simulink subsystem "PvtSubSys_VSM_ELK"  (R2020b)
settings: Solver=VariableStepAuto  StartTime=0.0  StopTime=10.0  RelTol=1e-3
values from neighbouring files (symbols this model uses):
  P_VSM_ELK_Curvature_R_Table : value not decoded    [ELK.sldd]
  P_VSM_ELK_Curvature_R_Table_Calibration : value not decoded    [ELK.sldd]
  P_VSM_ELK_Lane_Width_Table : value not decoded    [ELK.sldd]
  P_VSM_ELK_Lane_Width_Table_Calibration : value not decoded    [ELK.sldd]
  P_VSM_ELK_Lateral_Speed_Table : value not decoded    [ELK.sldd]
  P_VSM_ELK_Lateral_Speed_Table_Calibration : value not decoded    [ELK.sldd]
  P_VSM_ELK_OnComing_Lateral = 2.8    [ELK.sldd]
  P_VSM_ELK_OnComing_TTC = 3.0    [ELK.sldd]
  P_VSM_ELK_OverTaking_Lateral = 2.0    [ELK.sldd]
  P_VSM_ELK_OverTaking_TTC = 5.0    [ELK.sldd]
  P_VSM_ELK_Sensitive_Table : value not decoded    [ELK.sldd]
  P_VSM_ELK_Sensitive_Table_Calibration : value not decoded    [ELK.sldd]
  P_VSM_ELK_State_Absesp_enable = 1.0    [ELK.sldd]
  P_VSM_ELK_State_Accpedalrate_enable = 1.0    [ELK.sldd]
  P_VSM_ELK_State_Breakpressure_enable = 1.0    [ELK.sldd]
  P_VSM_ELK_State_DriverInputTrqValue_enable = 1.0    [ELK.sldd]
  P_VSM_ELK_State_Eps_enable = 1.0    [ELK.sldd]
  P_VSM_ELK_State_ESSSts_enable = 1.0    [ELK.sldd]
  P_VSM_ELK_State_Failsafe_enable = 1.0    [ELK.sldd]
  P_VSM_ELK_State_GEAR_enable = 1.0    [ELK.sldd]
  P_VSM_ELK_State_Handson_enable = 1.0    [ELK.sldd]
  P_VSM_ELK_State_Headingangle_enable = 1.0    [ELK.sldd]
  P_VSM_ELK_State_Lane_enable = 1.0    [ELK.sldd]
  P_VSM_ELK_State_LaneChange_enable = 1.0    [ELK.sldd]
  P_VSM_ELK_State_Lanecurve_enable = 1.0    [ELK.sldd]
  P_VSM_ELK_State_LateralAcce_enable = 1.0    [ELK.sldd]
  P_VSM_ELK_State_LongitudeAcc_enable = 1.0    [ELK.sldd]
  P_VSM_ELK_State_Overide_enable = 1.0    [ELK.sldd]
  P_VSM_ELK_State_Param_AngleOffset = 0.05    [ELK.sldd]
  P_VSM_ELK_State_Param_LaneTime : value not decoded    [ELK.sldd]
  P_VSM_ELK_State_Param_Oncoming = 0.55    [ELK.sldd]
  P_VSM_ELK_State_Param_OnTime : value not decoded    [ELK.sldd]
  P_VSM_ELK_State_Param_OutOffset = 0.15    [ELK.sldd]
  P_VSM_ELK_State_Param_Over = 0.55    [ELK.sldd]
  P_VSM_ELK_State_Param_OvTime : value not decoded    [ELK.sldd]
  P_VSM_ELK_State_Param_Speed : value not decoded    [ELK.sldd]
  P_VSM_ELK_State_SteerWheelAngle_enable = 1.0    [ELK.sldd]
  P_VSM_ELK_State_SteerWheelSpd_enable = 1.0    [ELK.sldd]
  P_VSM_ELK_State_TurnLight_enable = 1.0    [ELK.sldd]
  P_VSM_ELK_State_Vehspeed_enable = 1.0    [ELK.sldd]
  P_VSM_ELK_State_Yawsup_enable = 1.0    [ELK.sldd]
undefined symbols (not defined in the file or in its folder): ELKSTATE, P_Global_DxvRearBumper_m, P_Global_IEnvironment_RefPX_Front_Bumper, P_Global_IFV2Fwheel_Dx, P_Global_Vehicle_Length_m, P_Global_VehicleWidthMin_m, P_VSM_LSMC_SampleTime
libraries: simulink x167
(part 1 of 5)
settings Model: Creator=GW00133806  LastModifiedBy=GW00199575

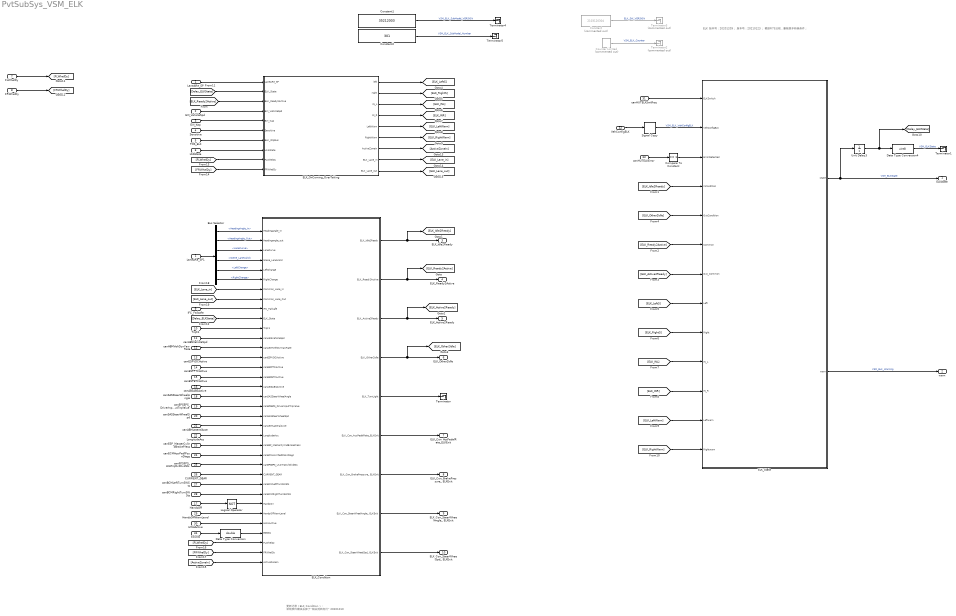
== system PvtSubSys_VSM_ELK ==
  note: 更新记录（ELK_Condition）：
      | 常规条件模块去掉了“相关则转向灯”
      | 20201010
  note: ELK
      | 版本号：20201209；
      | 版本号：20210123；
      | 根据R79法规，删除脱手转换条件；
  LaneARe_SP : Inport  OutDataTypeStr=Bus: LaneARe_SP
  EVI_VehicleSpd : Inport  Port=2  OutDataTypeStr=single
  EVI_Kap : Inport  Port=3  OutDataTypeStr=single
  Sensitive : Inport  Port=4  OutDataTypeStr=uint8
  TOS_ELK : Inport  Port=5  OutDataTypeStr=Bus: TOS_ELK_BUS  BusOutputAsStruct=on
  LKAState : Inport  Port=6  OutDataTypeStr=uint8
  FLWhelDy : Inport  Port=7  OutDataTypeStr=single
  FRWhelDy : Inport  Port=8  OutDataTypeStr=single
  IFC_Failsafe : Inport  Port=9  OutDataTypeStr=boolean
  TrqK1 : Inport  Port=10  OutDataTypeStr=single
  canABSVehicleSpd : Inport  Port=11  OutDataTypeStr=single
  canABMVehDynYawRate : Inport  Port=12  OutDataTypeStr=single
  canESPVDCActive : Inport  Port=13  OutDataTypeStr=boolean
  canESPPTCActive : Inport  Port=14  OutDataTypeStr=boolean
  canESPBTCActive : Inport  Port=15  OutDataTypeStr=boolean
  canABSABSActive : Inport  Port=16  OutDataTypeStr=boolean
  HandsOff : Inport  Port=17  OutDataTypeStr=boolean
  canSASSteerWheelAngle : Inport  Port=18  OutDataTypeStr=single
  canEPSEPS_DriverInputTrqValue : Inport  Port=19  OutDataTypeStr=single
  canSASSteerWheelSpd : Inport  Port=20  OutDataTypeStr=single
  canABMLateralAcce : Inport  Port=21  OutDataTypeStr=single
  LongitudeAcc : Inport  Port=22  OutDataTypeStr=single
  canESP_MasterCylindBrakePress : Inport  Port=23  OutDataTypeStr=single
  canECMAccrPedlPosnDiagc : Inport  Port=24  OutDataTypeStr=single
  canEPSEPS_LKATrqOvlDlvdSts : Inport  Port=25  OutDataTypeStr=uint8
  CURRENT_GEAR : Inport  Port=26  OutDataTypeStr=uint8
  canBCMLeftTurnSWSts : Inport  Port=27  OutDataTypeStr=boolean
  canBCMRightTurnSWSts : Inport  Port=28  OutDataTypeStr=boolean
  HandsOffWarnLevel : Inport  Port=29  OutDataTypeStr=uint8
  HWAActive : Inport  Port=30  OutDataTypeStr=boolean
  canHUTELKSwtReq : Inport  Port=31  OutDataTypeStr=boolean
  VehConfigELK : Inport  Port=32  OutDataTypeStr=uint8
  canHUTELKError : Inport  Port=33  OutDataTypeStr=uint8
  ESSSts : Inport  Port=34  OutDataTypeStr=uint8
  Bus Selector : BusSelector  OutputSignals=HeadingAngle_In,HeadingAngle_Out,LaneCurve,Scene_LaneValid,LeftChange,RightChange
  Compare To Constant : simulink/Logic and Bit Operations/Compare To Constant  relop===  const=1  OutDataTypeStr=boolean
  Constant : Constant  Commented=on  Value=2103120304  OutDataTypeStr=uint32
  Constant1 : Constant  Value=35212003  OutDataTypeStr=uint32
  Constant2 : Constant  Value=301  OutDataTypeStr=uint16
  Counter Limited : simulink/Sources/Counter Limited  Commented=on  uplimit=7  tsamp=-1
  Data Type Conversion : DataTypeConversion  OutDataTypeStr=double
  Data Type Conversion4 : DataTypeConversion  OutDataTypeStr=uint8
  ELK_Condition : Subsystem
  ELK_OnComing_OverTaking : Subsystem
  ELK_State : Stateflow chart  TreatAsAtomicUnit=on
  LaneARe_SP1 : InportShadow  OutDataTypeStr=Bus: LaneARe_SP
  Logical Operator : Logic  Operator=NOT  AllPortsSameDT=off  OutDataTypeStr=boolean
  Signal Copy : SignalConversion  OverrideOpt=off
  Terminator{,1,4..5} (4 alike) : Terminator
  Terminator2 : Terminator  Commented=on
  Terminator3 : Terminator  Commented=on
  Unit Delay3 : UnitDelay  InitialCondition=ELKSTATE.ELK_OFF  SampleTime=-1  HasFrameUpgradeWarning=on
  ELKstate : Outport  OutDataTypeStr=Enum: ELKSTATE
  warn : Outport  Port=2  OutDataTypeStr=single
  ELK_Idle2Ready : Outport  Port=3  OutDataTypeStr=boolean
  ELK_Ready2Active : Outport  Port=4  OutDataTypeStr=boolean
  ELK_Active2Ready : Outport  Port=5  OutDataTypeStr=boolean
  ELK_Other2Idle : Outport  Port=6  OutDataTypeStr=boolean
  ELK_Con_AccPedalRate_ELKExit : Outport  Port=7  OutDataTypeStr=boolean
  ELK_Con_BrakePressure_ ELKExit : Outport  Port=8  OutDataTypeStr=boolean
  ELK_Con_SteerWheelAngle_ ELKExit : Outport  Port=9  OutDataTypeStr=boolean
  ELK_Con_SteerWheelSpd_ ELKExit : Outport  Port=10  OutDataTypeStr=boolean
  wires:
  Constant2/1 -> Terminator5/1  "VSM_ELK_SubModel_Number"
  Constant1/1 -> Terminator4/1  "VSM_ELK_SubModel_VERSION"
  VehConfigELK/1 -> Signal Copy/1
  Bus Selector/6 -> ELK_Condition/6(RightChange)  "<RightChange>"
  Bus Selector/5 -> ELK_Condition/5(LeftChange)  "<LeftChange>"
  Data Type Conversion/1 -> ELK_Condition/32(ESSSts)
  [FLWhelDy] -> ELK_Condition/33(FLWhelDy)
  [FRWhelDy] -> ELK_Condition/34(FRWhelDy)
  [ActiveZoneIn] -> ELK_Condition/35(ActiveZoneIn)
  ELK_OnComing_OverTaking/7(ActiveZoneIn) -> [ActiveZoneIn]
  [FRWhelDy] -> ELK_OnComing_OverTaking/10(FRWhelDy)
  [FLWhelDy] -> ELK_OnComing_OverTaking/9(FLWhelDy)
  FRWhelDy/1 -> [FRWhelDy]
  FLWhelDy/1 -> [FLWhelDy]
  ESSSts/1 -> Data Type Conversion/1
  Logical Operator/1 -> ELK_Condition/29(HandsOn)
  ELK_Condition/9(ELK_Con_SteerWheelSpd_ ELKExit) -> ELK_Con_SteerWheelSpd_ ELKExit/1
  Unit Delay3/1 -> Data Type Conversion4/1, [Delay_ELKState]
  canABMLateralAcce/1 -> ELK_Condition/21(canABMLateralAcce)
  TrqK1/1 -> ELK_Condition/11(TrqK1)
  [ELK_RightWarn] -> ELK_State/13(Rightwarn)
  Signal Copy/1 -> ELK_State/2(VehConfigELK)  "VSM_ELK_VehConfigELK"
  [ELK_Ready2Active] -> ELK_State/6(Common)
  ELK_Condition/7(ELK_Con_BrakePressure_ ELKExit) -> ELK_Con_BrakePressure_ ELKExit/1
  canECMAccrPedlPosnDiagc/1 -> ELK_Condition/24(canECMAccrPedlPosnDiagc)
  LKAState/1 -> ELK_OnComing_OverTaking/8(LKAState)
  Bus Selector/1 -> ELK_Condition/1(Headingangle_In)  "<HeadingAngle_In>"
  canESPPTCActive/1 -> ELK_Condition/15(canESPPTCActive)
  canABSVehicleSpd/1 -> ELK_Condition/12(canABSVehicleSpd)
  ELK_OnComing_OverTaking/2("right ") -> [ELK_RightS]
  HandsOff/1 -> Logical Operator/1
  canESPBTCActive/1 -> ELK_Condition/16(canESPBTCActive)
  canHUTELKSwtReq/1 -> ELK_State/1(ELKSwitch)
  Bus Selector/4 -> ELK_Condition/4(Scene_LaneValid)  "<Scene_LaneValid>"
  Bus Selector/3 -> ELK_Condition/3(LaneCurve)  "<LaneCurve>"
  Bus Selector/2 -> ELK_Condition/2(Headingangle_out)  "<HeadingAngle_Out>"
  canSASSteerWheelAngle/1 -> ELK_Condition/18(canSASSteerWheelAngle)
  canESPVDCActive/1 -> ELK_Condition/14(canESPVDCActive)
  LaneARe_SP/1 -> ELK_OnComing_OverTaking/1(LaneARe_SP)
  [ELK_RightS] -> ELK_State/9(Right)
  Data Type Conversion4/1 -> Terminator1/1  "VSM_ELKState"
  ELK_Condition/1(ELK_Idle2Ready) -> [ELK_Idle2Ready], ELK_Idle2Ready/1
  IFC_Failsafe/1 -> ELK_Condition/9(IFC_Failsafe)
  canESP_MasterCylindBrakePress/1 -> ELK_Condition/23(canESP_MasterCylindBrakePress)
  Constant/1 -> Terminator3/1  "ELK_SW_VERSION"
  EVI_VehicleSpd/1 -> ELK_OnComing_OverTaking/4(EVI_VehicleSpd)
  Counter Limited/1 -> Terminator2/1  "VSM_ELK_Counter"
  ELK_Condition/5(ELK_TurnLight) -> Terminator/1
  ELK_OnComing_OverTaking/6(RightWarn) -> [ELK_RightWarn]
  ELK_Condition/6(ELK_Con_AccPedalRate_ELKExit) -> ELK_Con_AccPedalRate_ELKExit/1
  ELK_Condition/3(ELK_Active2Ready) -> [ELK_Active2Ready], ELK_Active2Ready/1
  ELK_OnComing_OverTaking/1("left ") -> [ELK_LeftS]
  ELK_OnComing_OverTaking/3(IN_L) -> [ELK_INL]
  canEPSEPS_DriverInputTrqValue/1 -> ELK_Condition/19(canEPSEPS_DriverInputTrqValue)
  TOS_ELK/1 -> ELK_OnComing_OverTaking/7(ELK_ObjBus)
  canSASSteerWheelSpd/1 -> ELK_Condition/20(canSASSteerWheelSpd)
  ELK_Condition/2(ELK_Ready2Active) -> [ELK_Ready2Active], ELK_Ready2Active/1
  canEPSEPS_LKATrqOvlDlvdSts/1 -> ELK_Condition/25(canEPSEPS_LKATrqOvlDlvdSts)
  Sensitive/1 -> ELK_OnComing_OverTaking/6(Sensitive)
  canBCMRightTurnSWSts/1 -> ELK_Condition/28(canBCMRightTurnSWSts)
  canHUTELKError/1 -> Compare To Constant/1
  canABMVehDynYawRate/1 -> ELK_Condition/13(canABMVehDynYawRate)
  canABSABSActive/1 -> ELK_Condition/17(canABSABSActive)
  LongitudeAcc/1 -> ELK_Condition/22(LongitudeAcc)
  CURRENT_GEAR/1 -> ELK_Condition/26(CURRENT_GEAR)
  [ELK_Active2Ready] -> ELK_State/7(Out_Common)
  ELK_Condition/4(ELK_Other2Idle) -> [ELK_Other2Idle], ELK_Other2Idle/1
  ELK_State/1(state) -> ELKstate/1, Unit Delay3/1  "VSM_ELKState"
  [ELK_INR] -> ELK_State/11(IN_R)
  canBCMLeftTurnSWSts/1 -> ELK_Condition/27(canBCMLeftTurnSWSts)
  ELK_OnComing_OverTaking/4(IN_R) -> [ELK_INR]
  [Delay_ELKState] -> ELK_Condition/10(ELK_State)
  [ELK_LeftWarn] -> ELK_State/12(Leftwarn)
  [ELK_Idle2Ready] -> ELK_State/4(InCondition)
  [ELK_LeftS] -> ELK_State/8(Left)
  [ELK_Other2Idle] -> ELK_State/5(OutCondition)
  ELK_OnComing_OverTaking/5(LeftWarn) -> [ELK_LeftWarn]
  [ELK_Ready2Active] -> ELK_OnComing_OverTaking/3(ELK_Ready2Active)
  [Delay_ELKState] -> ELK_OnComing_OverTaking/2(ELK_State)
  HandsOffWarnLevel/1 -> ELK_Condition/30(HandsOffWarnLevel)
  [ELK_INL] -> ELK_State/10(IN_L)
  ELK_State/2(warn) -> warn/1  "VSM_ELK_Warning"
  LaneARe_SP1/1 -> Bus Selector/1
  EVI_Kap/1 -> ELK_OnComing_OverTaking/5(EVI_Kap)
  ELK_Condition/8(ELK_Con_SteerWheelAngle_ ELKExit) -> ELK_Con_SteerWheelAngle_ ELKExit/1
  HWAActive/1 -> ELK_Condition/31(HWAActive)
  ELK_OnComing_OverTaking/8(ELK_Lane_in) -> [ELK_Lane_in]
  ELK_OnComing_OverTaking/9(ELK_Lane_out) -> [ELK_Lane_out]
  [ELK_Lane_in] -> ELK_Condition/7(Common_Lane_in)
  [ELK_Lane_out] -> ELK_Condition/8(Common_Lane_Out)
  Compare To Constant/1 -> ELK_State/3(ErrorDetected)
